simulink model "comunicacion_buena_ant"  (R2020b)
settings: Solver=FixedStepDiscrete  StartTime=0.0  StopTime=inf  FixedStep=0.005  RelTol=1e-3
undefined symbols (not defined in the file): Serial_Port, Standard_Devices
libraries: sldrtlib x2, simulink x2, cstblocks x1
settings Model: Creator=anton  LastModifiedBy=anton
settings RTWCC: Description=Simulink Desktop Real-Time  SystemTargetFile=sldrt.tlc  TemplateMakefile=sldrt.tmf  RTWCompilerOptimization=on
settings CodeAppCC: MaxIdLength=95
settings SimulinkDesktopRealTimeCC: TargetPreCompLibLocation=C:\Program Files\MATLAB\R2020b\toolbox\sldrt\lib\win64

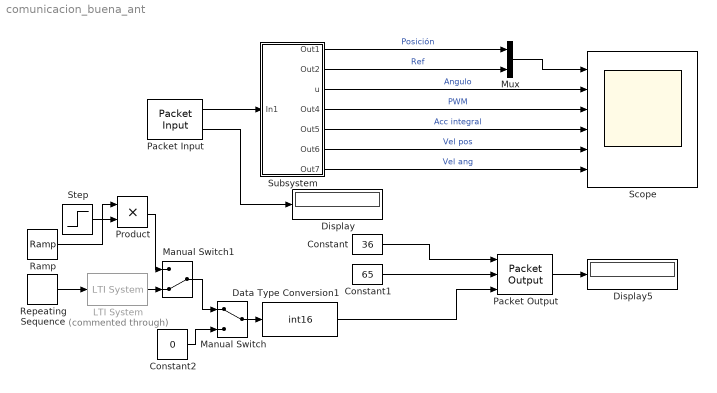
== system comunicacion_buena_ant ==
  Constant : Constant  Value=36  OutDataTypeStr=uint8
      mask Display: disp('$')
  Constant1 : Constant  Value=65  OutDataTypeStr=uint8
      mask Display: disp('A')
  Constant2 : Constant  Value=0
  Data Type Conversion1 : DataTypeConversion  OutDataTypeStr=int16
  Display : Display
  Display5 : Display
  LTI System : cstblocks/LTI System  Commented=through  sys=c2d(tf(1,[1 1]),0.005)  IC=[]
  Manual Switch : ManualSwitch
  Manual Switch1 : ManualSwitch  CurrentSetting=0
  Mux : Mux  Inputs=2
  Packet Input : sldrtlib/Packet Input  SampleTime=0.005  MaxMissedTicks=10  ShowMissedTicks=on  YieldWhenWaiting=off  DrvName=Standard_Devices/Serial_Port  DrvAddress=3  DrvOptions=[128000 8 0 0 0 0 0 0]  PacketSize=29  DataTypes={'29*uint8'}  ShowReady=off  ShowError=off  PacketID=1  ByteOrder=1  ShowTimestamp=off
      settings: AttributesFormatString=Serial Port [3]
  Packet Output : sldrtlib/Packet Output  SampleTime=0.1  MaxMissedTicks=10  ShowMissedTicks=on  YieldWhenWaiting=off  DrvName=Standard_Devices/Serial_Port  DrvAddress=3  DrvOptions=[128000 8 0 0 0 0 0 0]  PacketSize=4  DataTypes={'uint8','uint8','int16'}  ShowReady=off  ShowError=off  PacketID=1  ByteOrder=1  InitialValue=[]  FinalValue=[]
      settings: AttributesFormatString=Serial Port [3]
  Product : Product
  Ramp : simulink/Sources/Ramp  slope=72  start=15  InitialOutput=0
  Repeating Sequence : simulink/Sources/Repeating Sequence  rep_seq_t=[0 10 10.1 20 20.1 30 30.1 40 40.1]  rep_seq_y=[0 0 90 90 0 0 -90 -90 0]
  Scope : Scope  NumInputPorts=6
  Step : Step  Time=50  Before=1  After=0  SampleTime=0
  Subsystem : Subsystem
      mask Display: disp('Ordena')
  wires:
  Subsystem/1(Out1) -> Mux/1  "Posición"
  Subsystem/4(Out4) -> Scope/3  "PWM"
  Mux/1 -> Scope/1
  Subsystem/3(u) -> Scope/2  "Angulo"
  Subsystem/2(Out2) -> Mux/2  "Ref"
  Subsystem/7(Out7) -> Scope/6  "Vel ang"
  Subsystem/6(Out6) -> Scope/5  "Vel pos"
  Subsystem/5(Out5) -> Scope/4  "Acc integral"
  Packet Input/2 -> Display/1
  Data Type Conversion1/1 -> Packet Output/3
  Constant/1 -> Packet Output/1
  Constant1/1 -> Packet Output/2
  Packet Output/1 -> Display5/1
  Packet Input/1 -> Subsystem/1(In1)
  Repeating Sequence/1 -> LTI System/1
  Constant2/1 -> Manual Switch/2
  Manual Switch/1 -> Data Type Conversion1/1
  LTI System/1 -> Manual Switch1/2
  Manual Switch1/1 -> Manual Switch/1
  Ramp/1 -> Product/1
  Step/1 -> Product/2
  Product/1 -> Manual Switch1/1

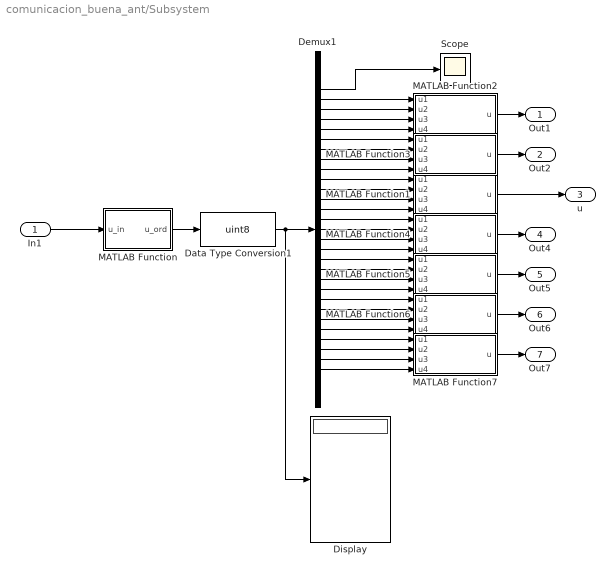
== system comunicacion_buena_ant/Subsystem ==
  In1 : Inport
  Data Type Conversion1 : DataTypeConversion  OutDataTypeStr=uint8
  Demux1 : Demux  Outputs=29
  Display : Display
  MATLAB Function : MATLAB Function  TreatAsAtomicUnit=on
  MATLAB Function1 : MATLAB Function  TreatAsAtomicUnit=on
  MATLAB Function2 : MATLAB Function  TreatAsAtomicUnit=on
  MATLAB Function3 : MATLAB Function  TreatAsAtomicUnit=on
  MATLAB Function4 : MATLAB Function  TreatAsAtomicUnit=on
  MATLAB Function5 : MATLAB Function  TreatAsAtomicUnit=on
  MATLAB Function6 : MATLAB Function  TreatAsAtomicUnit=on
  MATLAB Function7 : MATLAB Function  TreatAsAtomicUnit=on
  Scope : Scope
  Out1 : Outport
  Out2 : Outport  Port=2
  u : Outport  Port=3
  Out4 : Outport  Port=4
  Out5 : Outport  Port=5
  Out6 : Outport  Port=6
  Out7 : Outport  Port=7
  wires:
  In1/1 -> MATLAB Function/1(u_in)
  MATLAB Function/1(u_ord) -> Data Type Conversion1/1
  Demux1/26 -> MATLAB Function7/1(u1)
  Demux1/27 -> MATLAB Function7/2(u2)
  Demux1/28 -> MATLAB Function7/3(u3)
  Demux1/29 -> MATLAB Function7/4(u4)
  Demux1/22 -> MATLAB Function6/1(u1)
  Demux1/23 -> MATLAB Function6/2(u2)
  Demux1/24 -> MATLAB Function6/3(u3)
  Demux1/25 -> MATLAB Function6/4(u4)
  Demux1/18 -> MATLAB Function5/1(u1)
  Demux1/19 -> MATLAB Function5/2(u2)
  Demux1/21 -> MATLAB Function5/4(u4)
  Demux1/20 -> MATLAB Function5/3(u3)
  Demux1/16 -> MATLAB Function4/3(u3)
  Demux1/14 -> MATLAB Function4/1(u1)
  Demux1/15 -> MATLAB Function4/2(u2)
  Demux1/17 -> MATLAB Function4/4(u4)
  Demux1/12 -> MATLAB Function1/3(u3)
  Demux1/11 -> MATLAB Function1/2(u2)
  Demux1/13 -> MATLAB Function1/4(u4)
  Demux1/10 -> MATLAB Function1/1(u1)
  Demux1/8 -> MATLAB Function3/3(u3)
  Demux1/7 -> MATLAB Function3/2(u2)
  Demux1/9 -> MATLAB Function3/4(u4)
  Demux1/6 -> MATLAB Function3/1(u1)
  Demux1/4 -> MATLAB Function2/3(u3)
  Demux1/3 -> MATLAB Function2/2(u2)
  Demux1/5 -> MATLAB Function2/4(u4)
  Demux1/2 -> MATLAB Function2/1(u1)
  Demux1/1 -> Scope/1
  MATLAB Function2/1(u) -> Out1/1
  MATLAB Function3/1(u) -> Out2/1
  MATLAB Function1/1(u) -> u/1
  MATLAB Function4/1(u) -> Out4/1
  MATLAB Function5/1(u) -> Out5/1
  MATLAB Function6/1(u) -> Out6/1
  MATLAB Function7/1(u) -> Out7/1
  Data Type Conversion1/1 -> Display/1, Demux1/1

== matlab function comunicacion_buena_ant/Subsystem/MATLAB Function1 ==
  data: u1 input uint8 size=1; u output single size=1; u2 input uint8 size=1; u3 input uint8 size=1; u4 input uint8 size=1
function u= fcn(u1, u2, u3, u4)
%u=0;
% Byte1 = typecast(u1,'uint8');
% Byte2 = typecast(u2,'uint8');
% Byte3 = typecast(u3,'uint8');
% Byte4 = typecast(u4,'uint8');
%u = swapbytes(typecast([Byte1 Byte2 Byte3 Byte4],'single'));
u = typecast(typecast([u1 u2 u3 u4],'uint8'),'single');
end

== matlab function comunicacion_buena_ant/Subsystem/MATLAB Function ==
  data: u_in input; u_ord output
function u_ord = fcn(u_in)
inicio=1;
k=1;
for k=1:length(u_in)
    if u_in(k)==36
        inicio=k;
        break
    end
end
% Ordena
i=1; k=1;
u_ord = zeros(size(u_in));
for k=inicio:length(u_in)
    u_ord(i)=u_in(k);
    i=i+1;
end
for k=1:(inicio-1)
    u_ord(i)=u_in(k);
    i=i+1;
end

== matlab function comunicacion_buena_ant/Subsystem/MATLAB Function2 ==
  data: u1 input uint8 size=1; u output single size=1; u2 input uint8 size=1; u3 input uint8 size=1; u4 input uint8 size=1
function u= fcn(u1, u2, u3, u4)
%u=0;
% Byte1 = typecast(u1,'uint8');
% Byte2 = typecast(u2,'uint8');
% Byte3 = typecast(u3,'uint8');
% Byte4 = typecast(u4,'uint8');
%u = swapbytes(typecast([Byte1 Byte2 Byte3 Byte4],'single'));
u = typecast(typecast([u1 u2 u3 u4],'uint8'),'single');
end

== matlab function comunicacion_buena_ant/Subsystem/MATLAB Function3 ==
  data: u1 input uint8 size=1; u output single size=1; u2 input uint8 size=1; u3 input uint8 size=1; u4 input uint8 size=1
function u= fcn(u1, u2, u3, u4)
%u=0;
% Byte1 = typecast(u1,'uint8');
% Byte2 = typecast(u2,'uint8');
% Byte3 = typecast(u3,'uint8');
% Byte4 = typecast(u4,'uint8');
%u = swapbytes(typecast([Byte1 Byte2 Byte3 Byte4],'single'));
u = typecast(typecast([u1 u2 u3 u4],'uint8'),'single');
end

== matlab function comunicacion_buena_ant/Subsystem/MATLAB Function4 ==
  data: u1 input uint8 size=1; u output single size=1; u2 input uint8 size=1; u3 input uint8 size=1; u4 input uint8 size=1
function u= fcn(u1, u2, u3, u4)
%u=0;
% Byte1 = typecast(u1,'uint8');
% Byte2 = typecast(u2,'uint8');
% Byte3 = typecast(u3,'uint8');
% Byte4 = typecast(u4,'uint8');
%u = swapbytes(typecast([Byte1 Byte2 Byte3 Byte4],'single'));
u = typecast(typecast([u1 u2 u3 u4],'uint8'),'single');
end

== matlab function comunicacion_buena_ant/Subsystem/MATLAB Function5 ==
  data: u1 input uint8 size=1; u output single size=1; u2 input uint8 size=1; u3 input uint8 size=1; u4 input uint8 size=1
function u= fcn(u1, u2, u3, u4)
%u=0;
% Byte1 = typecast(u1,'uint8');
% Byte2 = typecast(u2,'uint8');
% Byte3 = typecast(u3,'uint8');
% Byte4 = typecast(u4,'uint8');
%u = swapbytes(typecast([Byte1 Byte2 Byte3 Byte4],'single'));
u = typecast(typecast([u1 u2 u3 u4],'uint8'),'single');
end

== matlab function comunicacion_buena_ant/Subsystem/MATLAB Function6 ==
  data: u1 input uint8 size=1; u output single size=1; u2 input uint8 size=1; u3 input uint8 size=1; u4 input uint8 size=1
function u= fcn(u1, u2, u3, u4)
%u=0;
% Byte1 = typecast(u1,'uint8');
% Byte2 = typecast(u2,'uint8');
% Byte3 = typecast(u3,'uint8');
% Byte4 = typecast(u4,'uint8');
%u = swapbytes(typecast([Byte1 Byte2 Byte3 Byte4],'single'));
u = typecast(typecast([u1 u2 u3 u4],'uint8'),'single');
end

== matlab function comunicacion_buena_ant/Subsystem/MATLAB Function7 ==
  data: u1 input uint8 size=1; u output single size=1; u2 input uint8 size=1; u3 input uint8 size=1; u4 input uint8 size=1
function u= fcn(u1, u2, u3, u4)
%u=0;
% Byte1 = typecast(u1,'uint8');
% Byte2 = typecast(u2,'uint8');
% Byte3 = typecast(u3,'uint8');
% Byte4 = typecast(u4,'uint8');
%u = swapbytes(typecast([Byte1 Byte2 Byte3 Byte4],'single'));
u = typecast(typecast([u1 u2 u3 u4],'uint8'),'single');
end
